simulink model "simular"  (R2020b)
settings: Solver=VariableStepAuto  StartTime=0.0  StopTime=15  RelTol=1e-3
settings Model: Creator=eriki  LastModifiedBy=eriki

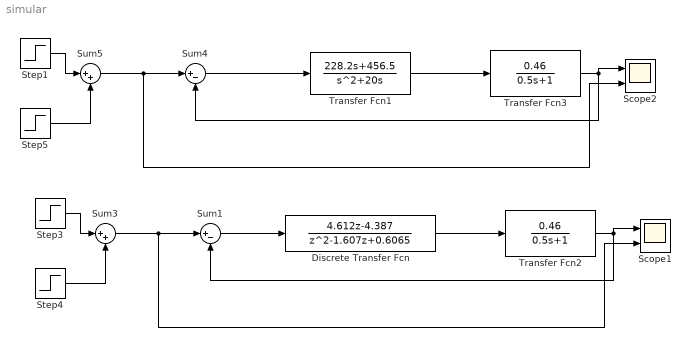
== system simular ==
  Discrete Transfer Fcn : DiscreteTransferFcn  Numerator=[4.612 -4.387]  Denominator=[1 -1.607 0.6065]  SampleTime=0.025
  Scope1 : Scope  NumInputPorts=2
  Scope2 : Scope  NumInputPorts=2
  Step1 : Step  Time=10  After=40  SampleTime=0
  Step3 : Step  Time=10  After=40  SampleTime=0
  Step4 : Step  After=40  SampleTime=0
  Step5 : Step  After=40  SampleTime=0
  Sum1 : Sum  Inputs=|+-
  Sum3 : Sum  Inputs=|++
  Sum4 : Sum  Inputs=|+-
  Sum5 : Sum  Inputs=|++
  Transfer Fcn1 : TransferFcn  Numerator=[228.2 456.5]  Denominator=[1 20 0]
  Transfer Fcn2 : TransferFcn  Numerator=0.46  Denominator=[0.5 1]
  Transfer Fcn3 : TransferFcn  Numerator=0.46  Denominator=[0.5 1]
  wires:
  Discrete Transfer Fcn/1 -> Transfer Fcn2/1
  Transfer Fcn2/1 -> Sum1/2, Scope1/1
  Sum1/1 -> Discrete Transfer Fcn/1
  Step3/1 -> Sum3/1
  Step4/1 -> Sum3/2
  Sum3/1 -> Sum1/1, Scope1/2
  Sum5/1 -> Sum4/1, Scope2/2
  Step5/1 -> Sum5/2
  Step1/1 -> Sum5/1
  Transfer Fcn1/1 -> Transfer Fcn3/1
  Transfer Fcn3/1 -> Sum4/2, Scope2/1
  Sum4/1 -> Transfer Fcn1/1
